simulink model "Lab2"  (R2021b)
settings: Solver=VariableStepAuto  StartTime=0.0  StopTime=9  RelTol=1e-3
libraries: simulink x1
settings Model: Creator=scott  LastModifiedBy=gajendrajayasekera
settings SolverCC: AlgebraicLoopSolver=TrustRegion
settings DebuggingCC: SFMachineParentedDataDiag=warning

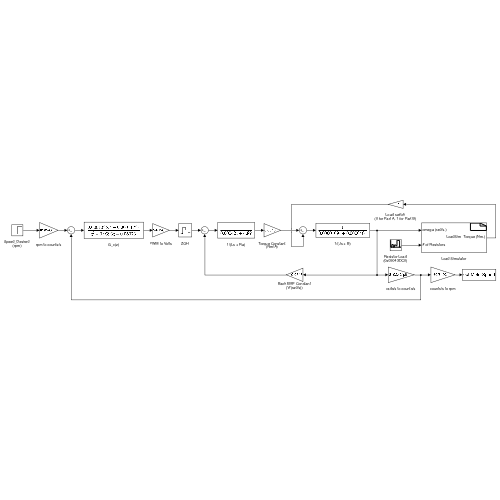
[thumbnail: Simulink's stored preview of the top-level diagram]
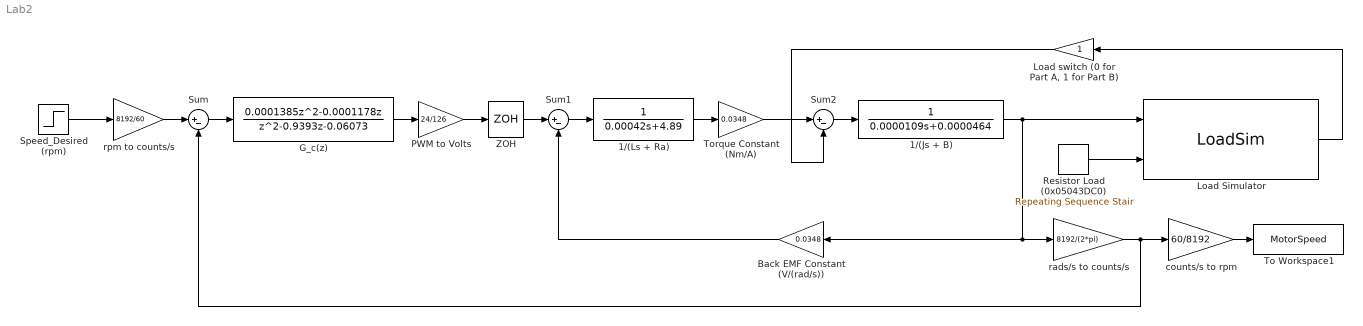
== system Lab2 ==
  " 1/(Js + B)" : TransferFcn  Denominator=[0.0000109 0.0000464]
  " 1/(Ls + Ra)" : TransferFcn  Denominator=[0.00042 4.89]
  " G_c(z)" : DiscreteTransferFcn  Numerator=[0.0001385 -0.0001178 0]  Denominator=[1 -0.9393 -0.06073]
  " Load Simulator" : S-Function  InitFcn=try, set_param(gcb,'FunctionName','LoadSim'), end  FunctionName=LoadSim  SFunctionModules=LoadSim_wrapper  SFunctionDeploymentMode=off  EnableBusSupport=off  mask(S-Function Builder){}
      mask help: Simulink:masks:SFunctionBuilder_MD
      mask init:
      | val = [[.9  0.75 0.75 1 1 .9 .9 1]',[1 1 0.75 0.75 .9 .9 1 .9]'];try , sys = get_param(gcb,'SfunBuilderFcnName');if isempty(sys), sys = get_param(gcb,'FunctionName'); end,catch, sys = get_param(gcb,'FunctionName'); end
      settings: CopyFcn=set_param(gcbh,'LinkStatus','none')  PreSaveFcn=try, set_param(gcb,'FunctionName','LoadSim'), end  OpenFcn=sfunctionwizard(gcbh)
      mask Display: plot(val(:,1),val(:,2)),disp(sys), port_label('input',1,'omega (rad/s.)'), port_label('input',2,'# of Resistors'), port_label('output',1,'Torque (Nm.)')
  " Load switch (0 for Part A, 1 for Part B)" : Gain
  " PWM to Volts" : Gain  Gain=24/126
  " Resistor Load (0x05043DC0)" : simulink/Sources/Repeating Sequence Stair  OutValues=[0 5 0 4 3 13 12 0].'  tsamp=0.006  OutMin=[]  OutMax=[]  OutDataTypeStr=double  OutputDataTypeScalingMode=double  OutDataType=fixdt(0,8)  ConRadixGroup=Best Precision: Vector-wise  OutScaling=2^-12
  " Speed_Desired (rpm)" : Step  Time=0  After=2000  SampleTime=0.006
  " Torque Constant (Nm/A)" : Gain  Gain=0.0348
  " ZOH" : ZeroOrderHold  SampleTime=-1
  " counts/s to rpm" : Gain  Gain=60/8192
  " rads/s to counts/s" : Gain  Gain=8192/(2*pi)
  " rpm to counts/s" : Gain  Gain=8192/60
  Back EMF Constant (V/(rad/s)) : Gain  Gain=0.0348
  Sum : Sum  Inputs=|+-
  Sum1 : Sum  Inputs=|+-
  Sum2 : Sum  Inputs=|+-
  To Workspace1 : ToWorkspace  VariableName=MotorSpeed  SaveFormat=Timeseries  SampleTime=-1
  wires:
  Sum1/1 -> " 1/(Ls + Ra)"/1
  " 1/(Ls + Ra)"/1 -> " Torque Constant (Nm/A)"/1
  " Torque Constant (Nm/A)"/1 -> Sum2/1
  " 1/(Js + B)"/1 -> " Load Simulator"/1, " rads/s to counts/s"/1, Back EMF Constant (V/(rad/s))/1
  " Load Simulator"/1 -> " Load switch (0 for Part A, 1 for Part B)"/1
  Back EMF Constant (V/(rad/s))/1 -> Sum1/2
  " rads/s to counts/s"/1 -> Sum/2, " counts/s to rpm"/1
  " ZOH"/1 -> Sum1/1
  " G_c(z)"/1 -> " PWM to Volts"/1
  " PWM to Volts"/1 -> " ZOH"/1
  Sum/1 -> " G_c(z)"/1
  " Speed_Desired (rpm)"/1 -> " rpm to counts/s"/1
  " rpm to counts/s"/1 -> Sum/1
  " Load switch (0 for Part A, 1 for Part B)"/1 -> Sum2/2
  " Resistor Load (0x05043DC0)"/1 -> " Load Simulator"/2
  Sum2/1 -> " 1/(Js + B)"/1
  " counts/s to rpm"/1 -> To Workspace1/1
